simulink model "Channelizer"  (R2026a)
settings: Solver=VariableStepAuto  StopTime=1e-5
InitFcn:
  | init;
values from neighbouring files (symbols this model uses):
  ch0_en = 0    [channelizer_demo_init.m]    (also in init.m)
  ch0_qam = 0    [channelizer_demo_init.m]    (also in init.m)
  ch0_swp = 0    [channelizer_demo_init.m]    (also in init.m)
  ch10_en = 0    [channelizer_demo_init.m]    (also in init.m)
  ch10_qam = 0    [channelizer_demo_init.m]    (also in init.m)
  ch10_swp = 0    [channelizer_demo_init.m]    (also in init.m)
  ch11_en = 0    [channelizer_demo_init.m]    (also in init.m)
  ch11_qam = 0    [channelizer_demo_init.m]    (also in init.m)
  ch11_swp = 0    [channelizer_demo_init.m]    (also in init.m)
  ch12_en = 0    [channelizer_demo_init.m]    (also in init.m)
  ch12_qam = 0    [channelizer_demo_init.m]    (also in init.m)
  ch12_swp = 0    [channelizer_demo_init.m]    (also in init.m)
  ch13_en = 0    [channelizer_demo_init.m]    (also in init.m)
  ch13_qam = 0    [channelizer_demo_init.m]    (also in init.m)
  ch13_swp = 0    [channelizer_demo_init.m]    (also in init.m)
  ch14_en = 0    [channelizer_demo_init.m]    (also in init.m)
  ch14_qam = 0    [channelizer_demo_init.m]    (also in init.m)
  ch14_swp = 0    [channelizer_demo_init.m]    (also in init.m)
  ch15_en = 0    [channelizer_demo_init.m]    (also in init.m)
  ch15_qam = 0    [channelizer_demo_init.m]    (also in init.m)
  ch15_swp = 0    [channelizer_demo_init.m]    (also in init.m)
  ch1_en = 1    [channelizer_demo_init.m]    (also in init.m)
  ch1_qam = 0    [channelizer_demo_init.m]    (also in init.m)
  ch1_swp = 0    [channelizer_demo_init.m]    (also in init.m)
  ch2_en = 1    [channelizer_demo_init.m]    (also in init.m)
  ch2_qam = 0    [channelizer_demo_init.m]    (also in init.m)
  ch2_swp = 0    [channelizer_demo_init.m]    (also in init.m)
  ch3_en = 0    [channelizer_demo_init.m]    (also in init.m)
  ch3_qam = 0    [channelizer_demo_init.m]    (also in init.m)
  ch3_swp = 0    [channelizer_demo_init.m]    (also in init.m)
  ch4_en = 0    [channelizer_demo_init.m]    (also in init.m)
  ch4_qam = 0    [channelizer_demo_init.m]    (also in init.m)
  ch4_swp = 0    [channelizer_demo_init.m]    (also in init.m)
  ch5_en = 1    [channelizer_demo_init.m]    (also in init.m)
  ch5_qam = 1    [channelizer_demo_init.m]    (also in init.m)
  ch5_swp = 0    [channelizer_demo_init.m]    (also in init.m)
  ch6_en = 1    [channelizer_demo_init.m]    (also in init.m)
  ch6_qam = 1    [channelizer_demo_init.m]    (also in init.m)
  ch6_swp = 0    [channelizer_demo_init.m]    (also in init.m)
  ch7_en = 0    [channelizer_demo_init.m]    (also in init.m)
  ch7_qam = 0    [channelizer_demo_init.m]    (also in init.m)
  ch7_swp = 0    [channelizer_demo_init.m]    (also in init.m)
  ch8_en = 0    [channelizer_demo_init.m]    (also in init.m)
  ch8_qam = 0    [channelizer_demo_init.m]    (also in init.m)
  ch8_swp = 0    [channelizer_demo_init.m]    (also in init.m)
  ch9_en = 0    [channelizer_demo_init.m]    (also in init.m)
  ch9_qam = 0    [channelizer_demo_init.m]    (also in init.m)
  ch9_swp = 0    [channelizer_demo_init.m]    (also in init.m)
  ch_filt_coef = 28 * ch_filt_coef / sum(ch_filt_coef(:))    [init.m]
  N = 2*1024    (= 2048)    [hil.m]    (also in init.m = 256)
  nvar = 0.01    [init.m]
  randph = 2*pi*rand(16,1)    [init.m]
  spec1_ch = 1    [channelizer_demo_init.m]    (also in init.m)
  spec2_ch = 2    [channelizer_demo_init.m]    (also in init.m)
  spec3_ch = 5    [channelizer_demo_init.m]    (also in init.m)
  spec4_ch = 6    [channelizer_demo_init.m]    (also in init.m)
  swp_rate0 = 0    [channelizer_demo_init.m]    (also in init.m)
  swp_rate1 = 0    [channelizer_demo_init.m]    (also in init.m)
  swp_rate10 = 0    [channelizer_demo_init.m]    (also in init.m)
  swp_rate11 = 0    [channelizer_demo_init.m]    (also in init.m)
  swp_rate12 = 0    [channelizer_demo_init.m]    (also in init.m)
  swp_rate13 = 0    [channelizer_demo_init.m]    (also in init.m)
  swp_rate14 = 0    [channelizer_demo_init.m]    (also in init.m)
  swp_rate15 = 0    [channelizer_demo_init.m]    (also in init.m)
  swp_rate2 = 0    [channelizer_demo_init.m]    (also in init.m)
  swp_rate3 = 0    [channelizer_demo_init.m]    (also in init.m)
  swp_rate4 = 0    [channelizer_demo_init.m]    (also in init.m)
  swp_rate5 = 0    [channelizer_demo_init.m]    (also in init.m)
  swp_rate6 = 0    [channelizer_demo_init.m]    (also in init.m)
  swp_rate7 = 0    [channelizer_demo_init.m]    (also in init.m)
  swp_rate8 = 0    [channelizer_demo_init.m]    (also in init.m)
  swp_rate9 = 0    [channelizer_demo_init.m]    (also in init.m)
  Ts = 16*(7/4)/8.75e9    (= 3.2e-09)    [init.m]
undefined symbols (not defined in the file or in its folder): Asymmetric, jsin, S, vsva2197, xcvc1902
libraries: aieUtilities x20, aieBasic x7, hlsBasic x4, aieDSP x2, vmcUtilities x1
(part 2 of 3)

== system Channelizer/DUT/AIE_FilterBank_SSR ==
  In1 : Inport
  PLIO1 : aieBasic/PLIO  PlioWidth=64  PlioFreqSpec=on  PlioFreq=625  ColLocation=0  channel=0  blockJsonConstraints=[]  deprecateConstraints=0
  PLIO48 : aieBasic/PLIO  PlioWidth=64  PlioFreqSpec=on  PlioFreq=625  ColLocation=0  channel=0  blockJsonConstraints=[]  deprecateConstraints=0
  run_i1 : aieBasic/AIE Class Kernel  KernelAllAttrs=|  PortNames={'sig_i'; 'sig_o'}  PortSerializedTypes={'{Q2{P{Tinput_stream{1{t{Scint16}}}}}}'; '{Q2{P{Toutput_stream{1{t{Scint16}}}}}}'}  PortWindowSizes={0.000000000000000000e+00; 0.000000000000000000e+00}  PortWindowMargins={0.000000000000000000e+00; 0.000000000000000000e+00}  PortSynchronicities={'auto', 'auto'}  PortSignalSizes={0.000000000000000000e+00; 1.024000000000000000e+03}  ClassTemplateSpecKind=implicit  ClassTemplateParamNames={'pattern'; 'NSAMP'}  ClassTemplateParamKinds={'nontype'; 'nontype'}  ClassTemplateParamTypes={'unsigned int'; 'unsigned int'}  ClassTemplateParamValues={'0', '2048'}  ClassCtorParamNames={'taps0_i'; 'taps1_i'}  ClassCtorParamSerializedTypes={'{R{C{Bi16}64}}'; '{R{C{Bi16}64}}'}  ClassCtorParamValues={'[0;2;-4;6;-13;54;-178;1985;-20;88;-287;1822;-22;100;-326;1570;2042;6;-4;2;259;-80;23;-8;569;-166;49;-9;911;-248;74;-14;-19;93;-307;1256;-14;74;-248;911;-9;49;-166;569;-8;23;-80;259;1256;-307;93;-19;1570;-326;100;-22;1822;-287;88;-20;1985;-178;54;-13;-8;23;-80;259;0;2;-4;6;-13;54;-178;1985;-20;88;-287;1822;1985;-178;54;-13;2042;6;-4;2;259;-80;23;-8;569;-166;49;-9;-22;100;-326;1570;-19;93;-307;1256;-14;74;-248;911;-9;49;-166;569;911;-248;74;-14;1256;-307;93;-19;1570;-326;100;-22;1822;-287;88;-20;-9;49;-166;569;-8;23;-80;259;0;2;-4;6;-13;54;-178;1985;1822;-287;88;-20;1985;-178;54;-13;2042;6;-4;2;259;-80;23;-8;-20;88;-287;1822;-22;100;-326;1570;-19;93;-307;1256;-14;74;-248;911;569;-166;49;-9;911;-248;74;-14;1256;-307;93;-19;1570;-326;100;-22;-14;74;-248;911;-9;49;-166;569;-8;23;-80;259;0;2;-4;6;1570;-326;100;-22;1822;-287;88;-20;1985;-178;54;-13;2042;6;-4;2;-13;54;-178;1985;-20;88;-287;1822;-22;100;-326;1570;-19;93;-307;1256;259;-80;23;-8;569;-166;49;-9;911;-248;74;-14;1256;-307;93;-19;-19;93;-307;1256;-14;74;-248;911;-9;49;-166;569;-8;23;-80;259;1256;-307;93;-19;1570;-326;100;-22;1822;-287;88;-20;1985;-178;54;-13;0;2;-4;6;-13;54;-178;1985;-20;88;-287;1822;-22;100;-326;1570;2042;6;-4;2;259;-80;23;-8;569;-166;49;-9;911;-248;74;-14;-22;100;-326;1570;-19;93;-307;1256;-14;74;-248;911;-9;49;-166;569;911;-248;74;-14;1256;-307;93;-19;1570;-326;100;-22;1822;-287;88;-20;-8;23;-80;259;0;2;-4;6;-13;54;-178;1985;-20;88;-287;1822;1985;-178;54;-13;2042;6;-4;2;259;-80;23;-8;569;-166;49;-9;-20;88;-287;1822;-22;100;-326;1570;-19;93;-307;1256;-14;74;-248;911;569;-166;49;-9;911;-248;74;-14;1256;-307;93;-19;1570;-326;100;-22;-9;49;-166;569;-8;23;-80;259;0;2;-4;6;-13;54;-178;1985;1822;-287;88;-20;1985;-178;54;-13;2042;6;-4;2;259;-80;23;-8;-13;54;-178;1985;-20;88;-287;1822;-22;100;-326;1570;-19;93;-307;1256;259;-80;23;-8;569;-166;49;-9;911;-248;74;-14;1256;-307;93;-19;-14;74;-248;911;-9;49;-166;569;-8;23;-80;259;0;2;-4;6;1570;-326;100;-22;1822;-287;88;-20;1985;-178;54;-13;2042;6;-4;2]', '[6;12;-40;124;-6;28;-95;2027;-17;74;-241;1916;-22;97;-314;1706;2027;-95;28;-6;124;-40;12;6;408;-123;36;-8;737;-209;62;-12;-21;99;-322;1419;-17;85;-281;1085;-12;62;-209;737;-8;36;-123;408;1085;-281;85;-17;1419;-322;99;-21;1706;-314;97;-22;1916;-241;74;-17;-8;36;-123;408;6;12;-40;124;-6;28;-95;2027;-17;74;-241;1916;1916;-241;74;-17;2027;-95;28;-6;124;-40;12;6;408;-123;36;-8;-22;97;-314;1706;-21;99;-322;1419;-17;85;-281;1085;-12;62;-209;737;737;-209;62;-12;1085;-281;85;-17;1419;-322;99;-21;1706;-314;97;-22;-12;62;-209;737;-8;36;-123;408;6;12;-40;124;-6;28;-95;2027;1706;-314;97;-22;1916;-241;74;-17;2027;-95;28;-6;124;-40;12;6;-17;74;-241;1916;-22;97;-314;1706;-21;99;-322;1419;-17;85;-281;1085;408;-123;36;-8;737;-209;62;-12;1085;-281;85;-17;1419;-322;99;-21;-17;85;-281;1085;-12;62;-209;737;-8;36;-123;408;6;12;-40;124;1419;-322;99;-21;1706;-314;97;-22;1916;-241;74;-17;2027;-95;28;-6;-6;28;-95;2027;-17;74;-241;1916;-22;97;-314;1706;-21;99;-322;1419;124;-40;12;6;408;-123;36;-8;737;-209;62;-12;1085;-281;85;-17;-21;99;-322;1419;-17;85;-281;1085;-12;62;-209;737;-8;36;-123;408;1085;-281;85;-17;1419;-322;99;-21;1706;-314;97;-22;1916;-241;74;-17;6;12;-40;124;-6;28;-95;2027;-17;74;-241;1916;-22;97;-314;1706;2027;-95;28;-6;124;-40;12;6;408;-123;36;-8;737;-209;62;-12;-22;97;-314;1706;-21;99;-322;1419;-17;85;-281;1085;-12;62;-209;737;737;-209;62;-12;1085;-281;85;-17;1419;-322;99;-21;1706;-314;97;-22;-8;36;-123;408;6;12;-40;124;-6;28;-95;2027;-17;74;-241;1916;1916;-241;74;-17;2027;-95;28;-6;124;-40;12;6;408;-123;36;-8;-17;74;-241;1916;-22;97;-314;1706;-21;99;-322;1419;-17;85;-281;1085;408;-123;36;-8;737;-209;62;-12;1085;-281;85;-17;1419;-322;99;-21;-12;62;-209;737;-8;36;-123;408;6;12;-40;124;-6;28;-95;2027;1706;-314;97;-22;1916;-241;74;-17;2027;-95;28;-6;124;-40;12;6;-6;28;-95;2027;-17;74;-241;1916;-22;97;-314;1706;-21;99;-322;1419;124;-40;12;6;408;-123;36;-8;737;-209;62;-12;1085;-281;85;-17;-17;85;-281;1085;-12;62;-209;737;-8;36;-123;408;6;12;-40;124;1419;-322;99;-21;1706;-314;97;-22;1916;-241;74;-17;2027;-95;28;-6]'}  ClassIndex=1  ClassCtorIndex=1  ClassTabVisible=on  ClassTemplateParamsVisible=on  ClassCtorDeclVisible=on  ClassCtorParamsVisible=on  FunctionTabVisible=on  PreSSR=8  isImport=false  FunctionDecl=|  PortAttrs={ 'input', 'sig_i', 'input_stream_cint16 * restrict', '', '0', '', ''; 'output', 'sig_o', 'output_stream_cint16 * restrict', '', '', '', '4*N' }  PortAttrsEnables={'off', 'off', 'off', 'off', 'off', 'off', 'off';'off', 'off', 'off', 'off', 'off', 'off', 'on'}  SampleTime=-1  ClassDeclTypeOptions=C[1 1]@t74@template < unsigned int pattern, unsigned int NSAMP > class polyphase_fir;  ClassDecl=template < unsigned int pattern, unsigned int NSAMP > class polyphase_fir;  ClassTemplateParams={ 'pattern', 'unsigned int', '[0; 1; 2; 3; 4; 5; 6; 7]'; 'NSAMP', 'unsigned int', 'NSAMP' }  ClassTemplateParamsEnables={'off', 'off', 'on';'off', 'off', 'on'}  ClassCtorDeclTypeOptions=C[1 1]@t69@polyphase_fir(int16 ( & taps0_i ) [ 64 ], int16 ( & taps1_i ) [ 64 ])  ClassCtorDecl=polyphase_fir(int16 ( & taps0_i ) [ 64 ], int16 ( & taps1_i ) [ 64 ])  ClassCtorParams={ 'taps0_i', 'int16 ( &) [ 64 ]', '[tile0_tapsA; tile1_tapsA; tile2_tapsA; tile3_tapsA; tile4_tapsA; tile5_tapsA; tile6_tapsA; tile7_tapsA]'; 'taps1_i', 'int16 ( &) [ 64 ]', '[tile0_tapsB; tile1_tapsB; tile2_tapsB; tile3_tapsB; tile4_tapsB; tile5_tapsB; tile6_tapsB; tile7_tapsB]' }  KernelHeaderFile=aie/polyphase_fir.h  KernelClassName=polyphase_fir  KernelFunction=run_i  KernelSourceFile=aie/polyphase_fir.cpp  KernelSearchPaths={}  PreProcOptions={}  ssr=filterbank_ssr  blockJsonConstraints=[]
      KernelAllAttrs=|
      | s[12;12;9;9;19;14;21;23;21;23;24;21;15;17;12;24;26;26;26;27;28;9;21;23;23;23;24;25;14;19;19;29]@FunctionNameDeclFileNamePortNamesPortTypesPortSerializedTypesPortDirectionsPortWindowSizeEnablesPortWindowMarginEnablesPortBufferSizeEnablesPortBufferMarginEnablesPortSynchronicityEnablesPortSignalSizeEnablesPortBufferSizesPortBufferMarginsFunctionDeclFunctionTemplateSpecKindFunctionTemplateParamNamesFunctionTemplateParamKindsFunctionTemplateParamTypesFunctionTemplateParamValuesFunctionTemplateParamEnablesClassDeclClassTemplateSpecKindClassTemplateParamNamesClassTemplateParamKindsClassTemplateParamTypesClassTemplateParamValuesClassTemplateParamEnablesClassCtorDeclsClassCtorParamNamesClassCtorParamTypesClassCtorParamSerializedTypes[1 1]@C[32 1]@t5@run_it25@../../aie/polyphase_fir.hC[2 1]@t5@sig_it5@sig_oC[2 1]@t30@input_stream_cint16 * restrictt31@output_stream_cint16 * restrictC[2 1]@t37@{Q2{P{Tinput_stream{1{t{Scint16}}}}}}t38@{Q2{P{Toutput_stream{1{t{Scint16}}}}}}C[2 1]@t5@inputt6@outputC[2 1]@l0@l0@C[2 1]@l0@l0@C[2 1]@l0@l0@C[2 1]@l0@l0@C[2 1]@l0@l0@C[2 1]@l0@l1@C[2 1]@nnC[2 1]@nnt158@template < unsigned int pattern, unsigned int NSAMP > 
      | void polyphase_fir::
      | run_i(input_stream_cint16 * restrict sig_i, output_stream_cint16 * restrict sig_o)t4@nonee[0 1]@e[0 1]@e[0 1]@e[0 1]@e[0 1]@t74@template < unsigned int pattern, unsigned int NSAMP > class polyphase_fir;t8@implicitC[2 1]@t7@patternt5@NSAMPC[2 1]@t7@nontypet7@nontypeC[2 1]@t12@unsigned intt12@unsigned intC[2 1]@nnC[2 1]@l1@l1@C[1 1]@t69@polyphase_fir(int16 ( & taps0_i ) [ 64 ], int16 ( & taps1_i ) [ 64 ])C[1 1]@C[2 1]@t7@taps0_it7@taps1_iC[1 1]@C[2 1]@t17@int16 ( &) [ 64 ]t17@int16 ( &) [ 64 ]C[1 1]@C[2 1]@t14@{R{C{Bi16}64}}t14@{R{C{Bi16}64}}
      FunctionDecl=|
      | template < unsigned int pattern, unsigned int NSAMP > 
      | void polyphase_fir::
      | run_i(input_stream_cint16 * restrict sig_i, output_stream_cint16 * restrict sig_o)
  Out1 : Outport
  wires:
  run_i1/1 -> PLIO1/1
  PLIO1/1 -> Out1/1
  PLIO48/1 -> run_i1/1
  In1/1 -> PLIO48/1

== system Channelizer/Wideband_Signal/Random QAM ==
  Add : Sum
  Constant1 : Constant  SampleTime=-1
  Constant17 : Constant  SampleTime=-1
  Gain1 : Gain  Gain=2
  Gain7 : Gain  Gain=2
  Gain9 : Gain  Gain=1/sqrt(10)
  Product : Product
  Real-Imag to Complex : RealImagToComplex
  Round : Rounding  Operator=round
  Round1 : Rounding  Operator=round
  Selector : Selector  InputPortWidth=32*N  IndexOptions=Index vector (dialog)  Indices=1:2:32*N  OutputSizes=1
  Selector1 : Selector  InputPortWidth=32*N  IndexOptions=Index vector (dialog)  Indices=2:2:32*N  OutputSizes=1
  Subtract1 : Sum  Inputs=+-
  Uniform Random Number : UniformRandomNumber  Minimum=0  Seed=round(2^32*rand(32*N,1))  SampleTime=Ts*N  VectorParams1D=off
  Uniform Random Number2 : UniformRandomNumber  Minimum=0  Seed=round(2^32*rand(32*N,1))  SampleTime=Ts*N  VectorParams1D=off
  Out1 : Outport
  wires:
  Gain7/1 -> Add/1
  Constant17/1 -> Add/2
  Real-Imag to Complex/1 -> Out1/1
  Gain9/1 -> Selector1/1, Selector/1
  Selector/1 -> Real-Imag to Complex/1
  Selector1/1 -> Real-Imag to Complex/2
  Round/1 -> Gain7/1
  Uniform Random Number/1 -> Round/1
  Uniform Random Number2/1 -> Round1/1
  Constant1/1 -> Subtract1/2
  Gain1/1 -> Subtract1/1
  Round1/1 -> Gain1/1
  Product/1 -> Gain9/1
  Add/1 -> Product/1
  Subtract1/1 -> Product/2

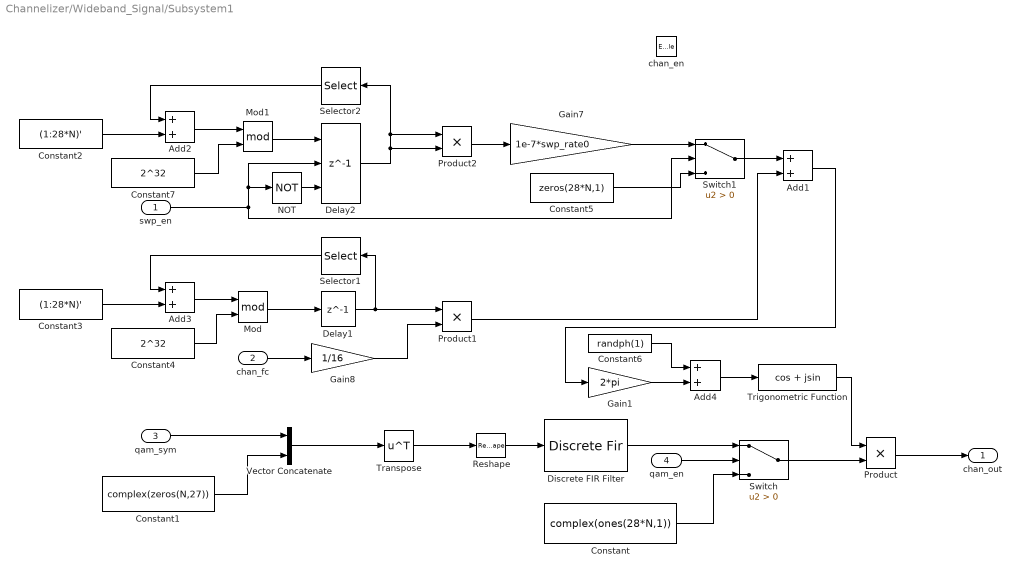
== system Channelizer/Wideband_Signal/Subsystem1 ==
  swp_en : Inport
  chan_fc : Inport  Port=2
  qam_sym : Inport  Port=3
  qam_en : Inport  Port=4
  chan_en : EnablePort
  Add{1..4} (4 alike) : Sum
  Constant : Constant  Value=complex(ones(28*N,1))  SampleTime=-1
  Constant1 : Constant  Value=complex(zeros(N,27))  VectorParams1D=off  SampleTime=-1
  Constant2 : Constant  Value=(1:28*N)'  SampleTime=-1
  Constant3 : Constant  Value=(1:28*N)'  SampleTime=-1
  Constant4 : Constant  Value=2^32  SampleTime=-1
  Constant5 : Constant  Value=zeros(28*N,1)  SampleTime=-1
  Constant6 : Constant  Value=randph(1)  SampleTime=-1
  Constant7 : Constant  Value=2^32  SampleTime=-1
  Delay1 : Delay  DelayLength=1  InitialCondition=(0:28*N-1)'
  Delay2 : Delay  DelayLength=1  InitialCondition=(1:28*N)'  ExternalReset=Falling  ShowEnablePort=on
      settings: InputPortMap=u0,e6,r5
  Discrete FIR Filter : DiscreteFir  Coefficients=ch_filt_coef  InputProcessing=Columns as channels (frame based)
  Gain1 : Gain  Gain=2*pi  OutDataTypeStr=double
  Gain7 : Gain  Gain=1e-7*swp_rate0  ParamDataTypeStr=double  OutDataTypeStr=double  SaturateOnIntegerOverflow=on
  Gain8 : Gain  Gain=1/16  OutDataTypeStr=double
  Mod : Math  Operator=mod
  Mod1 : Math  Operator=mod
  NOT : Logic  Operator=NOT  IconShape=distinctive  AllPortsSameDT=off  OutDataTypeStr=boolean
  Product : Product
  Product1 : Product
  Product2 : Product
  Reshape : Reshape
  Selector1 : Selector  InputPortWidth=28*N  IndexOptions=Index vector (dialog)  Indices=28*N  OutputSizes=1
  Selector2 : Selector  InputPortWidth=28*N  IndexOptions=Index vector (dialog)  Indices=28*N  OutputSizes=1
  Switch : Switch  Criteria=u2 > Threshold  SaturateOnIntegerOverflow=off  InputSameDT=off
  Switch1 : Switch  Criteria=u2 > Threshold  SaturateOnIntegerOverflow=off  InputSameDT=off
  Transpose : Math  Operator=transpose
  Trigonometric Function : Trigonometry  Operator=cos + jsin
  Vector Concatenate : Concatenate  Mode=Multidimensional array  ConcatenateDimension=2
  chan_out : Outport  OutputWhenDisabled=reset  InitialOutput=zeros(28*N,1)
  wires:
  Product/1 -> chan_out/1
  Switch/1 -> Product/2
  Discrete FIR Filter/1 -> Switch/1
  qam_en/1 -> Switch/2
  Constant/1 -> Switch/3
  Vector Concatenate/1 -> Transpose/1
  qam_sym/1 -> Vector Concatenate/1
  Constant1/1 -> Vector Concatenate/2
  Transpose/1 -> Reshape/1
  Reshape/1 -> Discrete FIR Filter/1
  Delay1/1 -> Product1/1, Selector1/1
  Selector1/1 -> Add3/1
  Constant3/1 -> Add3/2
  Mod/1 -> Delay1/1
  Add3/1 -> Mod/1
  Constant4/1 -> Mod/2
  Constant6/1 -> Add4/1
  Trigonometric Function/1 -> Product/1
  Add4/1 -> Trigonometric Function/1
  chan_fc/1 -> Gain8/1
  Gain8/1 -> Product1/2
  Gain1/1 -> Add4/2
  swp_en/1 -> NOT/1, Delay2/2, Switch1/2
  Constant5/1 -> Switch1/3
  Product2/1 -> Gain7/1
  Gain7/1 -> Switch1/1
  Switch1/1 -> Add1/1
  Product1/1 -> Add1/2
  Add1/1 -> Gain1/1
  Mod1/1 -> Delay2/1
  Constant2/1 -> Add2/2
  Selector2/1 -> Add2/1
  Delay2/1 -> Product2/1, Selector2/1, Product2/2
  Add2/1 -> Mod1/1
  Constant7/1 -> Mod1/2
  NOT/1 -> Delay2/3

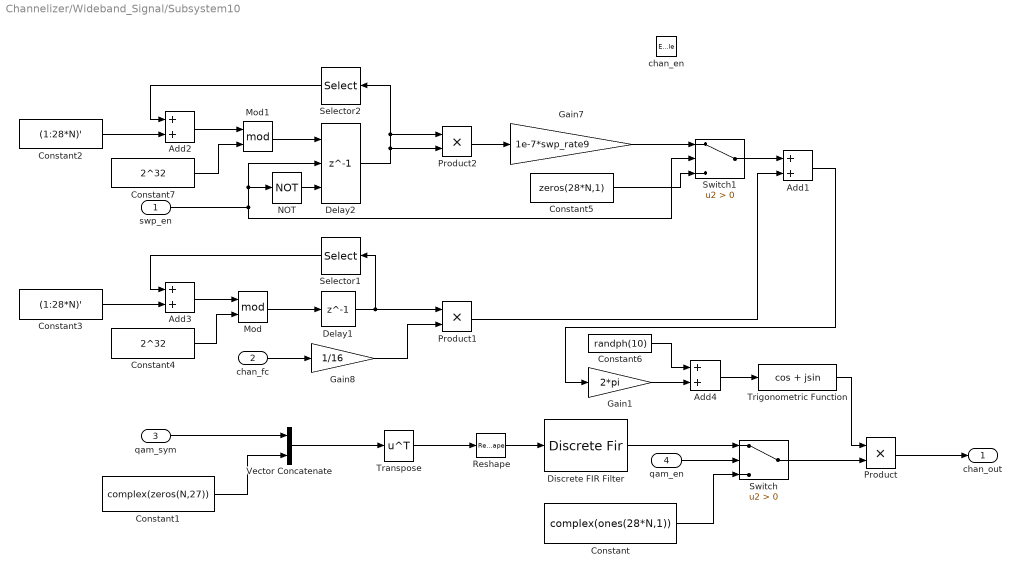
== system Channelizer/Wideband_Signal/Subsystem10 ==
  swp_en : Inport
  chan_fc : Inport  Port=2
  qam_sym : Inport  Port=3
  qam_en : Inport  Port=4
  chan_en : EnablePort
  Add{1..4} (4 alike) : Sum
  Constant : Constant  Value=complex(ones(28*N,1))  SampleTime=-1
  Constant1 : Constant  Value=complex(zeros(N,27))  VectorParams1D=off  SampleTime=-1
  Constant2 : Constant  Value=(1:28*N)'  SampleTime=-1
  Constant3 : Constant  Value=(1:28*N)'  SampleTime=-1
  Constant4 : Constant  Value=2^32  SampleTime=-1
  Constant5 : Constant  Value=zeros(28*N,1)  SampleTime=-1
  Constant6 : Constant  Value=randph(10)  SampleTime=-1
  Constant7 : Constant  Value=2^32  SampleTime=-1
  Delay1 : Delay  DelayLength=1  InitialCondition=(0:28*N-1)'
  Delay2 : Delay  DelayLength=1  InitialCondition=(1:28*N)'  ExternalReset=Falling  ShowEnablePort=on
      settings: InputPortMap=u0,e6,r5
  Discrete FIR Filter : DiscreteFir  Coefficients=ch_filt_coef  InputProcessing=Columns as channels (frame based)
  Gain1 : Gain  Gain=2*pi  OutDataTypeStr=double
  Gain7 : Gain  Gain=1e-7*swp_rate9  ParamDataTypeStr=double  OutDataTypeStr=double  SaturateOnIntegerOverflow=on
  Gain8 : Gain  Gain=1/16  OutDataTypeStr=double
  Mod : Math  Operator=mod
  Mod1 : Math  Operator=mod
  NOT : Logic  Operator=NOT  IconShape=distinctive  AllPortsSameDT=off  OutDataTypeStr=boolean
  Product : Product
  Product1 : Product
  Product2 : Product
  Reshape : Reshape
  Selector1 : Selector  InputPortWidth=28*N  IndexOptions=Index vector (dialog)  Indices=28*N  OutputSizes=1
  Selector2 : Selector  InputPortWidth=28*N  IndexOptions=Index vector (dialog)  Indices=28*N  OutputSizes=1
  Switch : Switch  Criteria=u2 > Threshold  SaturateOnIntegerOverflow=off  InputSameDT=off
  Switch1 : Switch  Criteria=u2 > Threshold  SaturateOnIntegerOverflow=off  InputSameDT=off
  Transpose : Math  Operator=transpose
  Trigonometric Function : Trigonometry  Operator=cos + jsin
  Vector Concatenate : Concatenate  Mode=Multidimensional array  ConcatenateDimension=2
  chan_out : Outport  OutputWhenDisabled=reset  InitialOutput=zeros(28*N,1)
  wires:
  Product/1 -> chan_out/1
  Switch/1 -> Product/2
  Discrete FIR Filter/1 -> Switch/1
  qam_en/1 -> Switch/2
  Constant/1 -> Switch/3
  Vector Concatenate/1 -> Transpose/1
  qam_sym/1 -> Vector Concatenate/1
  Constant1/1 -> Vector Concatenate/2
  Transpose/1 -> Reshape/1
  Reshape/1 -> Discrete FIR Filter/1
  Delay1/1 -> Product1/1, Selector1/1
  Selector1/1 -> Add3/1
  Constant3/1 -> Add3/2
  Mod/1 -> Delay1/1
  Add3/1 -> Mod/1
  Constant4/1 -> Mod/2
  Constant6/1 -> Add4/1
  Trigonometric Function/1 -> Product/1
  Add4/1 -> Trigonometric Function/1
  chan_fc/1 -> Gain8/1
  Gain8/1 -> Product1/2
  Gain1/1 -> Add4/2
  swp_en/1 -> NOT/1, Delay2/2, Switch1/2
  Constant5/1 -> Switch1/3
  Product2/1 -> Gain7/1
  Gain7/1 -> Switch1/1
  Switch1/1 -> Add1/1
  Product1/1 -> Add1/2
  Add1/1 -> Gain1/1
  Mod1/1 -> Delay2/1
  Constant2/1 -> Add2/2
  Selector2/1 -> Add2/1
  Delay2/1 -> Product2/1, Selector2/1, Product2/2
  Add2/1 -> Mod1/1
  Constant7/1 -> Mod1/2
  NOT/1 -> Delay2/3

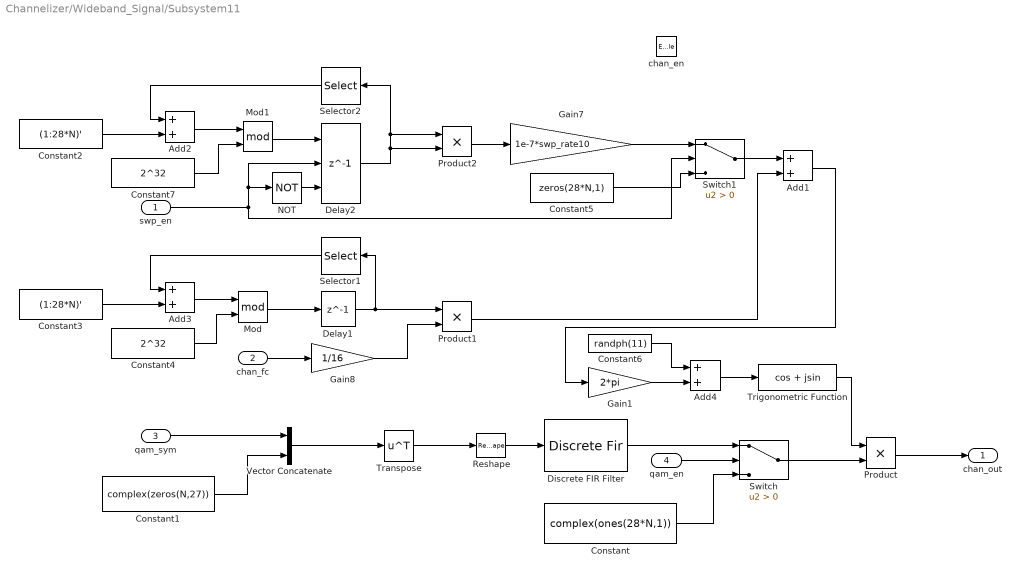
== system Channelizer/Wideband_Signal/Subsystem11 ==
  swp_en : Inport
  chan_fc : Inport  Port=2
  qam_sym : Inport  Port=3
  qam_en : Inport  Port=4
  chan_en : EnablePort
  Add{1..4} (4 alike) : Sum
  Constant : Constant  Value=complex(ones(28*N,1))  SampleTime=-1
  Constant1 : Constant  Value=complex(zeros(N,27))  VectorParams1D=off  SampleTime=-1
  Constant2 : Constant  Value=(1:28*N)'  SampleTime=-1
  Constant3 : Constant  Value=(1:28*N)'  SampleTime=-1
  Constant4 : Constant  Value=2^32  SampleTime=-1
  Constant5 : Constant  Value=zeros(28*N,1)  SampleTime=-1
  Constant6 : Constant  Value=randph(11)  SampleTime=-1
  Constant7 : Constant  Value=2^32  SampleTime=-1
  Delay1 : Delay  DelayLength=1  InitialCondition=(0:28*N-1)'
  Delay2 : Delay  DelayLength=1  InitialCondition=(1:28*N)'  ExternalReset=Falling  ShowEnablePort=on
      settings: InputPortMap=u0,e6,r5
  Discrete FIR Filter : DiscreteFir  Coefficients=ch_filt_coef  InputProcessing=Columns as channels (frame based)
  Gain1 : Gain  Gain=2*pi  OutDataTypeStr=double
  Gain7 : Gain  Gain=1e-7*swp_rate10  ParamDataTypeStr=double  OutDataTypeStr=double  SaturateOnIntegerOverflow=on
  Gain8 : Gain  Gain=1/16  OutDataTypeStr=double
  Mod : Math  Operator=mod
  Mod1 : Math  Operator=mod
  NOT : Logic  Operator=NOT  IconShape=distinctive  AllPortsSameDT=off  OutDataTypeStr=boolean
  Product : Product
  Product1 : Product
  Product2 : Product
  Reshape : Reshape
  Selector1 : Selector  InputPortWidth=28*N  IndexOptions=Index vector (dialog)  Indices=28*N  OutputSizes=1
  Selector2 : Selector  InputPortWidth=28*N  IndexOptions=Index vector (dialog)  Indices=28*N  OutputSizes=1
  Switch : Switch  Criteria=u2 > Threshold  SaturateOnIntegerOverflow=off  InputSameDT=off
  Switch1 : Switch  Criteria=u2 > Threshold  SaturateOnIntegerOverflow=off  InputSameDT=off
  Transpose : Math  Operator=transpose
  Trigonometric Function : Trigonometry  Operator=cos + jsin
  Vector Concatenate : Concatenate  Mode=Multidimensional array  ConcatenateDimension=2
  chan_out : Outport  OutputWhenDisabled=reset  InitialOutput=zeros(28*N,1)
  wires:
  Product/1 -> chan_out/1
  Switch/1 -> Product/2
  Discrete FIR Filter/1 -> Switch/1
  qam_en/1 -> Switch/2
  Constant/1 -> Switch/3
  Vector Concatenate/1 -> Transpose/1
  qam_sym/1 -> Vector Concatenate/1
  Constant1/1 -> Vector Concatenate/2
  Transpose/1 -> Reshape/1
  Reshape/1 -> Discrete FIR Filter/1
  Delay1/1 -> Product1/1, Selector1/1
  Selector1/1 -> Add3/1
  Constant3/1 -> Add3/2
  Mod/1 -> Delay1/1
  Add3/1 -> Mod/1
  Constant4/1 -> Mod/2
  Constant6/1 -> Add4/1
  Trigonometric Function/1 -> Product/1
  Add4/1 -> Trigonometric Function/1
  chan_fc/1 -> Gain8/1
  Gain8/1 -> Product1/2
  Gain1/1 -> Add4/2
  swp_en/1 -> NOT/1, Delay2/2, Switch1/2
  Constant5/1 -> Switch1/3
  Product2/1 -> Gain7/1
  Gain7/1 -> Switch1/1
  Switch1/1 -> Add1/1
  Product1/1 -> Add1/2
  Add1/1 -> Gain1/1
  Mod1/1 -> Delay2/1
  Constant2/1 -> Add2/2
  Selector2/1 -> Add2/1
  Delay2/1 -> Product2/1, Selector2/1, Product2/2
  Add2/1 -> Mod1/1
  Constant7/1 -> Mod1/2
  NOT/1 -> Delay2/3

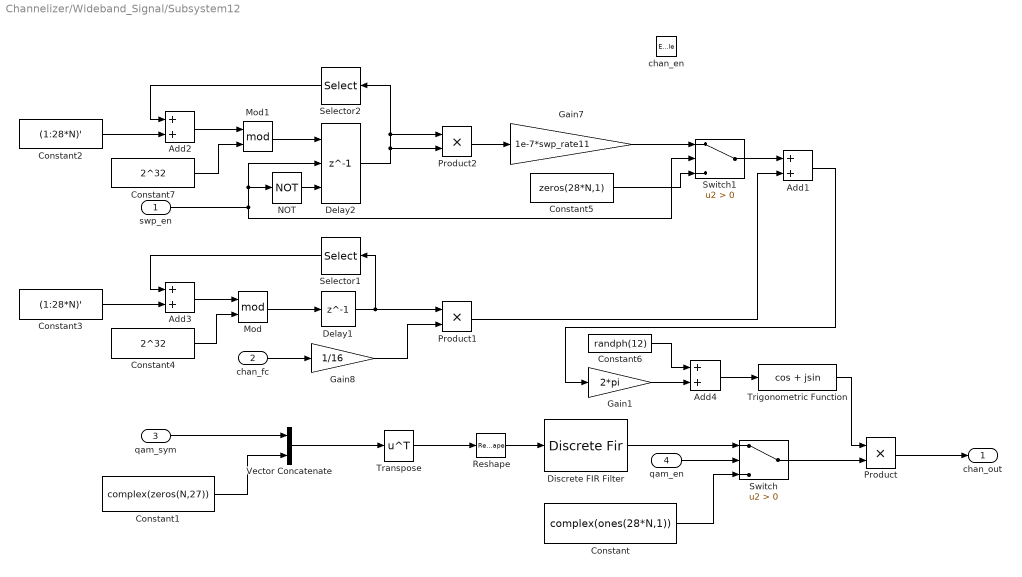
== system Channelizer/Wideband_Signal/Subsystem12 ==
  swp_en : Inport
  chan_fc : Inport  Port=2
  qam_sym : Inport  Port=3
  qam_en : Inport  Port=4
  chan_en : EnablePort
  Add{1..4} (4 alike) : Sum
  Constant : Constant  Value=complex(ones(28*N,1))  SampleTime=-1
  Constant1 : Constant  Value=complex(zeros(N,27))  VectorParams1D=off  SampleTime=-1
  Constant2 : Constant  Value=(1:28*N)'  SampleTime=-1
  Constant3 : Constant  Value=(1:28*N)'  SampleTime=-1
  Constant4 : Constant  Value=2^32  SampleTime=-1
  Constant5 : Constant  Value=zeros(28*N,1)  SampleTime=-1
  Constant6 : Constant  Value=randph(12)  SampleTime=-1
  Constant7 : Constant  Value=2^32  SampleTime=-1
  Delay1 : Delay  DelayLength=1  InitialCondition=(0:28*N-1)'
  Delay2 : Delay  DelayLength=1  InitialCondition=(1:28*N)'  ExternalReset=Falling  ShowEnablePort=on
      settings: InputPortMap=u0,e6,r5
  Discrete FIR Filter : DiscreteFir  Coefficients=ch_filt_coef  InputProcessing=Columns as channels (frame based)
  Gain1 : Gain  Gain=2*pi  OutDataTypeStr=double
  Gain7 : Gain  Gain=1e-7*swp_rate11  ParamDataTypeStr=double  OutDataTypeStr=double  SaturateOnIntegerOverflow=on
  Gain8 : Gain  Gain=1/16  OutDataTypeStr=double
  Mod : Math  Operator=mod
  Mod1 : Math  Operator=mod
  NOT : Logic  Operator=NOT  IconShape=distinctive  AllPortsSameDT=off  OutDataTypeStr=boolean
  Product : Product
  Product1 : Product
  Product2 : Product
  Reshape : Reshape
  Selector1 : Selector  InputPortWidth=28*N  IndexOptions=Index vector (dialog)  Indices=28*N  OutputSizes=1
  Selector2 : Selector  InputPortWidth=28*N  IndexOptions=Index vector (dialog)  Indices=28*N  OutputSizes=1
  Switch : Switch  Criteria=u2 > Threshold  SaturateOnIntegerOverflow=off  InputSameDT=off
  Switch1 : Switch  Criteria=u2 > Threshold  SaturateOnIntegerOverflow=off  InputSameDT=off
  Transpose : Math  Operator=transpose
  Trigonometric Function : Trigonometry  Operator=cos + jsin
  Vector Concatenate : Concatenate  Mode=Multidimensional array  ConcatenateDimension=2
  chan_out : Outport  OutputWhenDisabled=reset  InitialOutput=zeros(28*N,1)
  wires:
  Product/1 -> chan_out/1
  Switch/1 -> Product/2
  Discrete FIR Filter/1 -> Switch/1
  qam_en/1 -> Switch/2
  Constant/1 -> Switch/3
  Vector Concatenate/1 -> Transpose/1
  qam_sym/1 -> Vector Concatenate/1
  Constant1/1 -> Vector Concatenate/2
  Transpose/1 -> Reshape/1
  Reshape/1 -> Discrete FIR Filter/1
  Delay1/1 -> Product1/1, Selector1/1
  Selector1/1 -> Add3/1
  Constant3/1 -> Add3/2
  Mod/1 -> Delay1/1
  Add3/1 -> Mod/1
  Constant4/1 -> Mod/2
  Constant6/1 -> Add4/1
  Trigonometric Function/1 -> Product/1
  Add4/1 -> Trigonometric Function/1
  chan_fc/1 -> Gain8/1
  Gain8/1 -> Product1/2
  Gain1/1 -> Add4/2
  swp_en/1 -> NOT/1, Delay2/2, Switch1/2
  Constant5/1 -> Switch1/3
  Product2/1 -> Gain7/1
  Gain7/1 -> Switch1/1
  Switch1/1 -> Add1/1
  Product1/1 -> Add1/2
  Add1/1 -> Gain1/1
  Mod1/1 -> Delay2/1
  Constant2/1 -> Add2/2
  Selector2/1 -> Add2/1
  Delay2/1 -> Product2/1, Selector2/1, Product2/2
  Add2/1 -> Mod1/1
  Constant7/1 -> Mod1/2
  NOT/1 -> Delay2/3

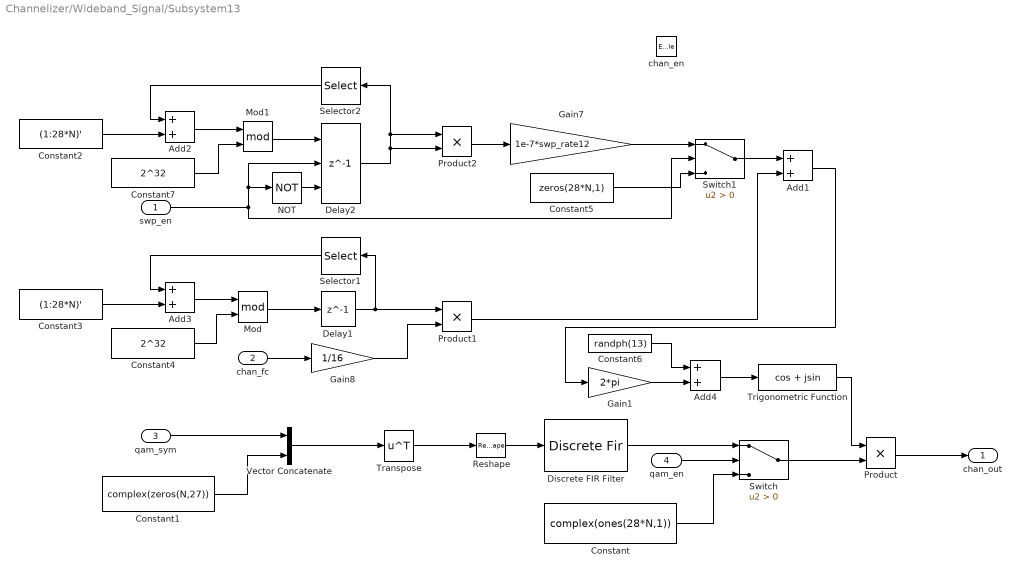
== system Channelizer/Wideband_Signal/Subsystem13 ==
  swp_en : Inport
  chan_fc : Inport  Port=2
  qam_sym : Inport  Port=3
  qam_en : Inport  Port=4
  chan_en : EnablePort
  Add{1..4} (4 alike) : Sum
  Constant : Constant  Value=complex(ones(28*N,1))  SampleTime=-1
  Constant1 : Constant  Value=complex(zeros(N,27))  VectorParams1D=off  SampleTime=-1
  Constant2 : Constant  Value=(1:28*N)'  SampleTime=-1
  Constant3 : Constant  Value=(1:28*N)'  SampleTime=-1
  Constant4 : Constant  Value=2^32  SampleTime=-1
  Constant5 : Constant  Value=zeros(28*N,1)  SampleTime=-1
  Constant6 : Constant  Value=randph(13)  SampleTime=-1
  Constant7 : Constant  Value=2^32  SampleTime=-1
  Delay1 : Delay  DelayLength=1  InitialCondition=(0:28*N-1)'
  Delay2 : Delay  DelayLength=1  InitialCondition=(1:28*N)'  ExternalReset=Falling  ShowEnablePort=on
      settings: InputPortMap=u0,e6,r5
  Discrete FIR Filter : DiscreteFir  Coefficients=ch_filt_coef  InputProcessing=Columns as channels (frame based)
  Gain1 : Gain  Gain=2*pi  OutDataTypeStr=double
  Gain7 : Gain  Gain=1e-7*swp_rate12  ParamDataTypeStr=double  OutDataTypeStr=double  SaturateOnIntegerOverflow=on
  Gain8 : Gain  Gain=1/16  OutDataTypeStr=double
  Mod : Math  Operator=mod
  Mod1 : Math  Operator=mod
  NOT : Logic  Operator=NOT  IconShape=distinctive  AllPortsSameDT=off  OutDataTypeStr=boolean
  Product : Product
  Product1 : Product
  Product2 : Product
  Reshape : Reshape
  Selector1 : Selector  InputPortWidth=28*N  IndexOptions=Index vector (dialog)  Indices=28*N  OutputSizes=1
  Selector2 : Selector  InputPortWidth=28*N  IndexOptions=Index vector (dialog)  Indices=28*N  OutputSizes=1
  Switch : Switch  Criteria=u2 > Threshold  SaturateOnIntegerOverflow=off  InputSameDT=off
  Switch1 : Switch  Criteria=u2 > Threshold  SaturateOnIntegerOverflow=off  InputSameDT=off
  Transpose : Math  Operator=transpose
  Trigonometric Function : Trigonometry  Operator=cos + jsin
  Vector Concatenate : Concatenate  Mode=Multidimensional array  ConcatenateDimension=2
  chan_out : Outport  OutputWhenDisabled=reset  InitialOutput=zeros(28*N,1)
  wires:
  Product/1 -> chan_out/1
  Switch/1 -> Product/2
  Discrete FIR Filter/1 -> Switch/1
  qam_en/1 -> Switch/2
  Constant/1 -> Switch/3
  Vector Concatenate/1 -> Transpose/1
  qam_sym/1 -> Vector Concatenate/1
  Constant1/1 -> Vector Concatenate/2
  Transpose/1 -> Reshape/1
  Reshape/1 -> Discrete FIR Filter/1
  Delay1/1 -> Product1/1, Selector1/1
  Selector1/1 -> Add3/1
  Constant3/1 -> Add3/2
  Mod/1 -> Delay1/1
  Add3/1 -> Mod/1
  Constant4/1 -> Mod/2
  Constant6/1 -> Add4/1
  Trigonometric Function/1 -> Product/1
  Add4/1 -> Trigonometric Function/1
  chan_fc/1 -> Gain8/1
  Gain8/1 -> Product1/2
  Gain1/1 -> Add4/2
  swp_en/1 -> NOT/1, Delay2/2, Switch1/2
  Constant5/1 -> Switch1/3
  Product2/1 -> Gain7/1
  Gain7/1 -> Switch1/1
  Switch1/1 -> Add1/1
  Product1/1 -> Add1/2
  Add1/1 -> Gain1/1
  Mod1/1 -> Delay2/1
  Constant2/1 -> Add2/2
  Selector2/1 -> Add2/1
  Delay2/1 -> Product2/1, Selector2/1, Product2/2
  Add2/1 -> Mod1/1
  Constant7/1 -> Mod1/2
  NOT/1 -> Delay2/3

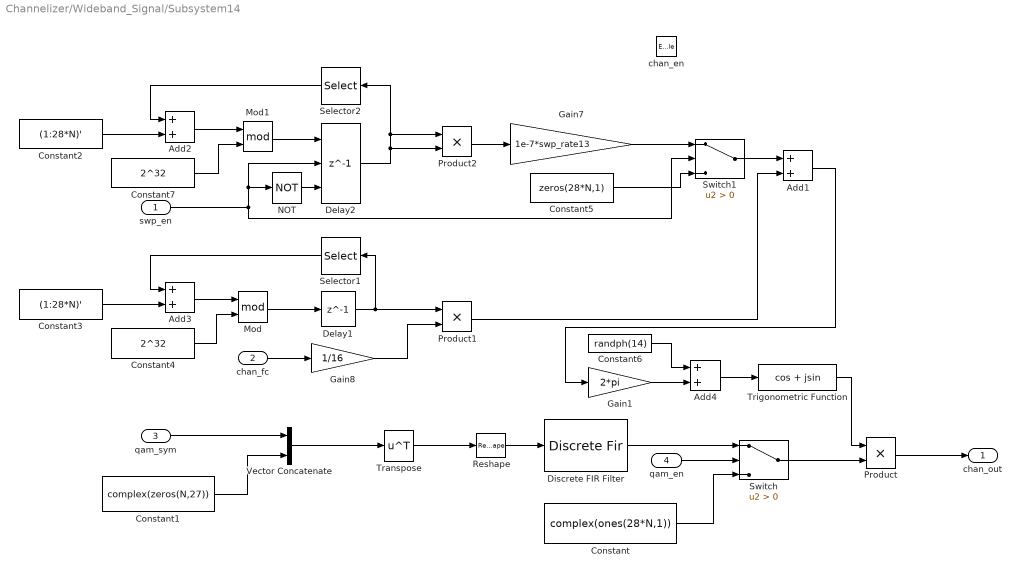
== system Channelizer/Wideband_Signal/Subsystem14 ==
  swp_en : Inport
  chan_fc : Inport  Port=2
  qam_sym : Inport  Port=3
  qam_en : Inport  Port=4
  chan_en : EnablePort
  Add{1..4} (4 alike) : Sum
  Constant : Constant  Value=complex(ones(28*N,1))  SampleTime=-1
  Constant1 : Constant  Value=complex(zeros(N,27))  VectorParams1D=off  SampleTime=-1
  Constant2 : Constant  Value=(1:28*N)'  SampleTime=-1
  Constant3 : Constant  Value=(1:28*N)'  SampleTime=-1
  Constant4 : Constant  Value=2^32  SampleTime=-1
  Constant5 : Constant  Value=zeros(28*N,1)  SampleTime=-1
  Constant6 : Constant  Value=randph(14)  SampleTime=-1
  Constant7 : Constant  Value=2^32  SampleTime=-1
  Delay1 : Delay  DelayLength=1  InitialCondition=(0:28*N-1)'
  Delay2 : Delay  DelayLength=1  InitialCondition=(1:28*N)'  ExternalReset=Falling  ShowEnablePort=on
      settings: InputPortMap=u0,e6,r5
  Discrete FIR Filter : DiscreteFir  Coefficients=ch_filt_coef  InputProcessing=Columns as channels (frame based)
  Gain1 : Gain  Gain=2*pi  OutDataTypeStr=double
  Gain7 : Gain  Gain=1e-7*swp_rate13  ParamDataTypeStr=double  OutDataTypeStr=double  SaturateOnIntegerOverflow=on
  Gain8 : Gain  Gain=1/16  OutDataTypeStr=double
  Mod : Math  Operator=mod
  Mod1 : Math  Operator=mod
  NOT : Logic  Operator=NOT  IconShape=distinctive  AllPortsSameDT=off  OutDataTypeStr=boolean
  Product : Product
  Product1 : Product
  Product2 : Product
  Reshape : Reshape
  Selector1 : Selector  InputPortWidth=28*N  IndexOptions=Index vector (dialog)  Indices=28*N  OutputSizes=1
  Selector2 : Selector  InputPortWidth=28*N  IndexOptions=Index vector (dialog)  Indices=28*N  OutputSizes=1
  Switch : Switch  Criteria=u2 > Threshold  SaturateOnIntegerOverflow=off  InputSameDT=off
  Switch1 : Switch  Criteria=u2 > Threshold  SaturateOnIntegerOverflow=off  InputSameDT=off
  Transpose : Math  Operator=transpose
  Trigonometric Function : Trigonometry  Operator=cos + jsin
  Vector Concatenate : Concatenate  Mode=Multidimensional array  ConcatenateDimension=2
  chan_out : Outport  OutputWhenDisabled=reset  InitialOutput=zeros(28*N,1)
  wires:
  Product/1 -> chan_out/1
  Switch/1 -> Product/2
  Discrete FIR Filter/1 -> Switch/1
  qam_en/1 -> Switch/2
  Constant/1 -> Switch/3
  Vector Concatenate/1 -> Transpose/1
  qam_sym/1 -> Vector Concatenate/1
  Constant1/1 -> Vector Concatenate/2
  Transpose/1 -> Reshape/1
  Reshape/1 -> Discrete FIR Filter/1
  Delay1/1 -> Product1/1, Selector1/1
  Selector1/1 -> Add3/1
  Constant3/1 -> Add3/2
  Mod/1 -> Delay1/1
  Add3/1 -> Mod/1
  Constant4/1 -> Mod/2
  Constant6/1 -> Add4/1
  Trigonometric Function/1 -> Product/1
  Add4/1 -> Trigonometric Function/1
  chan_fc/1 -> Gain8/1
  Gain8/1 -> Product1/2
  Gain1/1 -> Add4/2
  swp_en/1 -> NOT/1, Delay2/2, Switch1/2
  Constant5/1 -> Switch1/3
  Product2/1 -> Gain7/1
  Gain7/1 -> Switch1/1
  Switch1/1 -> Add1/1
  Product1/1 -> Add1/2
  Add1/1 -> Gain1/1
  Mod1/1 -> Delay2/1
  Constant2/1 -> Add2/2
  Selector2/1 -> Add2/1
  Delay2/1 -> Product2/1, Selector2/1, Product2/2
  Add2/1 -> Mod1/1
  Constant7/1 -> Mod1/2
  NOT/1 -> Delay2/3

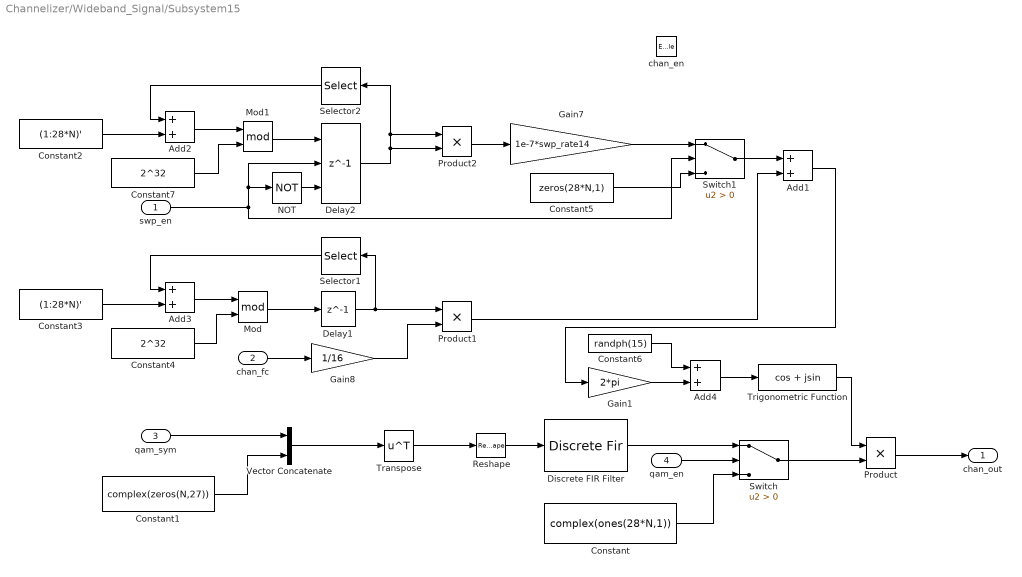
== system Channelizer/Wideband_Signal/Subsystem15 ==
  swp_en : Inport
  chan_fc : Inport  Port=2
  qam_sym : Inport  Port=3
  qam_en : Inport  Port=4
  chan_en : EnablePort
  Add{1..4} (4 alike) : Sum
  Constant : Constant  Value=complex(ones(28*N,1))  SampleTime=-1
  Constant1 : Constant  Value=complex(zeros(N,27))  VectorParams1D=off  SampleTime=-1
  Constant2 : Constant  Value=(1:28*N)'  SampleTime=-1
  Constant3 : Constant  Value=(1:28*N)'  SampleTime=-1
  Constant4 : Constant  Value=2^32  SampleTime=-1
  Constant5 : Constant  Value=zeros(28*N,1)  SampleTime=-1
  Constant6 : Constant  Value=randph(15)  SampleTime=-1
  Constant7 : Constant  Value=2^32  SampleTime=-1
  Delay1 : Delay  DelayLength=1  InitialCondition=(0:28*N-1)'
  Delay2 : Delay  DelayLength=1  InitialCondition=(1:28*N)'  ExternalReset=Falling  ShowEnablePort=on
      settings: InputPortMap=u0,e6,r5
  Discrete FIR Filter : DiscreteFir  Coefficients=ch_filt_coef  InputProcessing=Columns as channels (frame based)
  Gain1 : Gain  Gain=2*pi  OutDataTypeStr=double
  Gain7 : Gain  Gain=1e-7*swp_rate14  ParamDataTypeStr=double  OutDataTypeStr=double  SaturateOnIntegerOverflow=on
  Gain8 : Gain  Gain=1/16  OutDataTypeStr=double
  Mod : Math  Operator=mod
  Mod1 : Math  Operator=mod
  NOT : Logic  Operator=NOT  IconShape=distinctive  AllPortsSameDT=off  OutDataTypeStr=boolean
  Product : Product
  Product1 : Product
  Product2 : Product
  Reshape : Reshape
  Selector1 : Selector  InputPortWidth=28*N  IndexOptions=Index vector (dialog)  Indices=28*N  OutputSizes=1
  Selector2 : Selector  InputPortWidth=28*N  IndexOptions=Index vector (dialog)  Indices=28*N  OutputSizes=1
  Switch : Switch  Criteria=u2 > Threshold  SaturateOnIntegerOverflow=off  InputSameDT=off
  Switch1 : Switch  Criteria=u2 > Threshold  SaturateOnIntegerOverflow=off  InputSameDT=off
  Transpose : Math  Operator=transpose
  Trigonometric Function : Trigonometry  Operator=cos + jsin
  Vector Concatenate : Concatenate  Mode=Multidimensional array  ConcatenateDimension=2
  chan_out : Outport  OutputWhenDisabled=reset  InitialOutput=zeros(28*N,1)
  wires:
  Product/1 -> chan_out/1
  Switch/1 -> Product/2
  Discrete FIR Filter/1 -> Switch/1
  qam_en/1 -> Switch/2
  Constant/1 -> Switch/3
  Vector Concatenate/1 -> Transpose/1
  qam_sym/1 -> Vector Concatenate/1
  Constant1/1 -> Vector Concatenate/2
  Transpose/1 -> Reshape/1
  Reshape/1 -> Discrete FIR Filter/1
  Delay1/1 -> Product1/1, Selector1/1
  Selector1/1 -> Add3/1
  Constant3/1 -> Add3/2
  Mod/1 -> Delay1/1
  Add3/1 -> Mod/1
  Constant4/1 -> Mod/2
  Constant6/1 -> Add4/1
  Trigonometric Function/1 -> Product/1
  Add4/1 -> Trigonometric Function/1
  chan_fc/1 -> Gain8/1
  Gain8/1 -> Product1/2
  Gain1/1 -> Add4/2
  swp_en/1 -> NOT/1, Delay2/2, Switch1/2
  Constant5/1 -> Switch1/3
  Product2/1 -> Gain7/1
  Gain7/1 -> Switch1/1
  Switch1/1 -> Add1/1
  Product1/1 -> Add1/2
  Add1/1 -> Gain1/1
  Mod1/1 -> Delay2/1
  Constant2/1 -> Add2/2
  Selector2/1 -> Add2/1
  Delay2/1 -> Product2/1, Selector2/1, Product2/2
  Add2/1 -> Mod1/1
  Constant7/1 -> Mod1/2
  NOT/1 -> Delay2/3

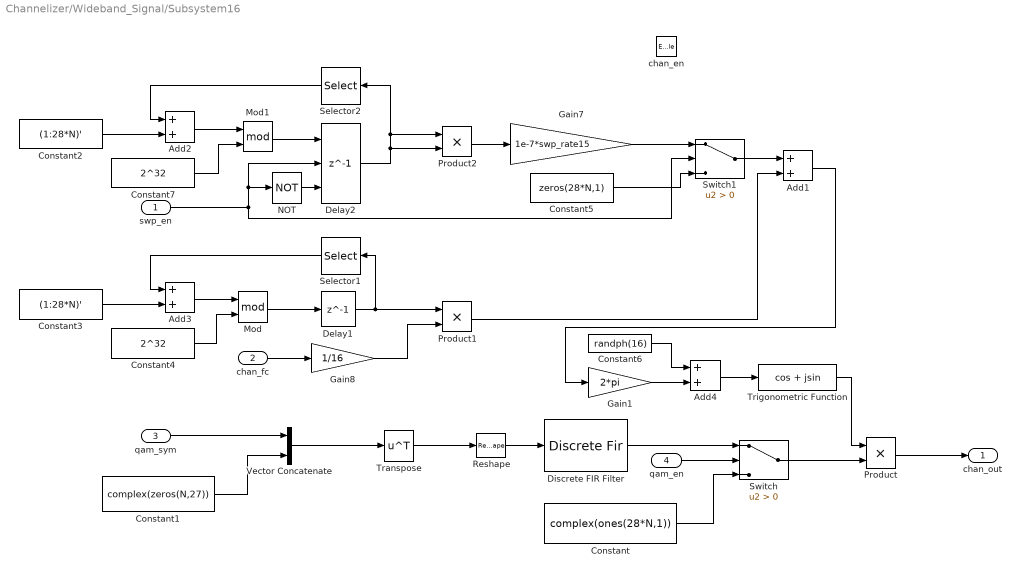
== system Channelizer/Wideband_Signal/Subsystem16 ==
  swp_en : Inport
  chan_fc : Inport  Port=2
  qam_sym : Inport  Port=3
  qam_en : Inport  Port=4
  chan_en : EnablePort
  Add{1..4} (4 alike) : Sum
  Constant : Constant  Value=complex(ones(28*N,1))  SampleTime=-1
  Constant1 : Constant  Value=complex(zeros(N,27))  VectorParams1D=off  SampleTime=-1
  Constant2 : Constant  Value=(1:28*N)'  SampleTime=-1
  Constant3 : Constant  Value=(1:28*N)'  SampleTime=-1
  Constant4 : Constant  Value=2^32  SampleTime=-1
  Constant5 : Constant  Value=zeros(28*N,1)  SampleTime=-1
  Constant6 : Constant  Value=randph(16)  SampleTime=-1
  Constant7 : Constant  Value=2^32  SampleTime=-1
  Delay1 : Delay  DelayLength=1  InitialCondition=(0:28*N-1)'
  Delay2 : Delay  DelayLength=1  InitialCondition=(1:28*N)'  ExternalReset=Falling  ShowEnablePort=on
      settings: InputPortMap=u0,e6,r5
  Discrete FIR Filter : DiscreteFir  Coefficients=ch_filt_coef  InputProcessing=Columns as channels (frame based)
  Gain1 : Gain  Gain=2*pi  OutDataTypeStr=double
  Gain7 : Gain  Gain=1e-7*swp_rate15  ParamDataTypeStr=double  OutDataTypeStr=double  SaturateOnIntegerOverflow=on
  Gain8 : Gain  Gain=1/16  OutDataTypeStr=double
  Mod : Math  Operator=mod
  Mod1 : Math  Operator=mod
  NOT : Logic  Operator=NOT  IconShape=distinctive  AllPortsSameDT=off  OutDataTypeStr=boolean
  Product : Product
  Product1 : Product
  Product2 : Product
  Reshape : Reshape
  Selector1 : Selector  InputPortWidth=28*N  IndexOptions=Index vector (dialog)  Indices=28*N  OutputSizes=1
  Selector2 : Selector  InputPortWidth=28*N  IndexOptions=Index vector (dialog)  Indices=28*N  OutputSizes=1
  Switch : Switch  Criteria=u2 > Threshold  SaturateOnIntegerOverflow=off  InputSameDT=off
  Switch1 : Switch  Criteria=u2 > Threshold  SaturateOnIntegerOverflow=off  InputSameDT=off
  Transpose : Math  Operator=transpose
  Trigonometric Function : Trigonometry  Operator=cos + jsin
  Vector Concatenate : Concatenate  Mode=Multidimensional array  ConcatenateDimension=2
  chan_out : Outport  OutputWhenDisabled=reset  InitialOutput=zeros(28*N,1)
  wires:
  Product/1 -> chan_out/1
  Switch/1 -> Product/2
  Discrete FIR Filter/1 -> Switch/1
  qam_en/1 -> Switch/2
  Constant/1 -> Switch/3
  Vector Concatenate/1 -> Transpose/1
  qam_sym/1 -> Vector Concatenate/1
  Constant1/1 -> Vector Concatenate/2
  Transpose/1 -> Reshape/1
  Reshape/1 -> Discrete FIR Filter/1
  Delay1/1 -> Product1/1, Selector1/1
  Selector1/1 -> Add3/1
  Constant3/1 -> Add3/2
  Mod/1 -> Delay1/1
  Add3/1 -> Mod/1
  Constant4/1 -> Mod/2
  Constant6/1 -> Add4/1
  Trigonometric Function/1 -> Product/1
  Add4/1 -> Trigonometric Function/1
  chan_fc/1 -> Gain8/1
  Gain8/1 -> Product1/2
  Gain1/1 -> Add4/2
  swp_en/1 -> NOT/1, Delay2/2, Switch1/2
  Constant5/1 -> Switch1/3
  Product2/1 -> Gain7/1
  Gain7/1 -> Switch1/1
  Switch1/1 -> Add1/1
  Product1/1 -> Add1/2
  Add1/1 -> Gain1/1
  Mod1/1 -> Delay2/1
  Constant2/1 -> Add2/2
  Selector2/1 -> Add2/1
  Delay2/1 -> Product2/1, Selector2/1, Product2/2
  Add2/1 -> Mod1/1
  Constant7/1 -> Mod1/2
  NOT/1 -> Delay2/3

== system Channelizer/Wideband_Signal/Subsystem2 ==
  swp_en : Inport
  chan_fc : Inport  Port=2
  qam_sym : Inport  Port=3
  qam_en : Inport  Port=4
  chan_en : EnablePort
  Add{1..4} (4 alike) : Sum
  Constant : Constant  Value=complex(ones(28*N,1))  SampleTime=-1
  Constant1 : Constant  Value=complex(zeros(N,27))  VectorParams1D=off  SampleTime=-1
  Constant2 : Constant  Value=(1:28*N)'  SampleTime=-1
  Constant3 : Constant  Value=(1:28*N)'  SampleTime=-1
  Constant4 : Constant  Value=2^32  SampleTime=-1
  Constant5 : Constant  Value=zeros(28*N,1)  SampleTime=-1
  Constant6 : Constant  Value=randph(2)  SampleTime=-1
  Constant7 : Constant  Value=2^32  SampleTime=-1
  Delay1 : Delay  DelayLength=1  InitialCondition=(0:28*N-1)'
  Delay2 : Delay  DelayLength=1  InitialCondition=(1:28*N)'  ExternalReset=Falling  ShowEnablePort=on
      settings: InputPortMap=u0,e6,r5
  Discrete FIR Filter : DiscreteFir  Coefficients=ch_filt_coef  InputProcessing=Columns as channels (frame based)
  Gain1 : Gain  Gain=2*pi  OutDataTypeStr=double
  Gain7 : Gain  Gain=1e-7*swp_rate1  ParamDataTypeStr=double  OutDataTypeStr=double  SaturateOnIntegerOverflow=on
  Gain8 : Gain  Gain=1/16  OutDataTypeStr=double
  Mod : Math  Operator=mod
  Mod1 : Math  Operator=mod
  NOT : Logic  Operator=NOT  IconShape=distinctive  AllPortsSameDT=off  OutDataTypeStr=boolean
  Product : Product
  Product1 : Product
  Product2 : Product
  Reshape : Reshape
  Selector1 : Selector  InputPortWidth=28*N  IndexOptions=Index vector (dialog)  Indices=28*N  OutputSizes=1
  Selector2 : Selector  InputPortWidth=28*N  IndexOptions=Index vector (dialog)  Indices=28*N  OutputSizes=1
  Switch : Switch  Criteria=u2 > Threshold  SaturateOnIntegerOverflow=off  InputSameDT=off
  Switch1 : Switch  Criteria=u2 > Threshold  SaturateOnIntegerOverflow=off  InputSameDT=off
  Transpose : Math  Operator=transpose
  Trigonometric Function : Trigonometry  Operator=cos + jsin
  Vector Concatenate : Concatenate  Mode=Multidimensional array  ConcatenateDimension=2
  chan_out : Outport  OutputWhenDisabled=reset  InitialOutput=zeros(28*N,1)
  wires:
  Product/1 -> chan_out/1
  Switch/1 -> Product/2
  Discrete FIR Filter/1 -> Switch/1
  qam_en/1 -> Switch/2
  Constant/1 -> Switch/3
  Vector Concatenate/1 -> Transpose/1
  qam_sym/1 -> Vector Concatenate/1
  Constant1/1 -> Vector Concatenate/2
  Transpose/1 -> Reshape/1
  Reshape/1 -> Discrete FIR Filter/1
  Delay1/1 -> Product1/1, Selector1/1
  Selector1/1 -> Add3/1
  Constant3/1 -> Add3/2
  Mod/1 -> Delay1/1
  Add3/1 -> Mod/1
  Constant4/1 -> Mod/2
  Constant6/1 -> Add4/1
  Trigonometric Function/1 -> Product/1
  Add4/1 -> Trigonometric Function/1
  chan_fc/1 -> Gain8/1
  Gain8/1 -> Product1/2
  Gain1/1 -> Add4/2
  swp_en/1 -> NOT/1, Delay2/2, Switch1/2
  Constant5/1 -> Switch1/3
  Product2/1 -> Gain7/1
  Gain7/1 -> Switch1/1
  Switch1/1 -> Add1/1
  Product1/1 -> Add1/2
  Add1/1 -> Gain1/1
  Mod1/1 -> Delay2/1
  Constant2/1 -> Add2/2
  Selector2/1 -> Add2/1
  Delay2/1 -> Product2/1, Selector2/1, Product2/2
  Add2/1 -> Mod1/1
  Constant7/1 -> Mod1/2
  NOT/1 -> Delay2/3

== system Channelizer/Wideband_Signal/Subsystem3 ==
  swp_en : Inport
  chan_fc : Inport  Port=2
  qam_sym : Inport  Port=3
  qam_en : Inport  Port=4
  chan_en : EnablePort
  Add{1..4} (4 alike) : Sum
  Constant : Constant  Value=complex(ones(28*N,1))  SampleTime=-1
  Constant1 : Constant  Value=complex(zeros(N,27))  VectorParams1D=off  SampleTime=-1
  Constant2 : Constant  Value=(1:28*N)'  SampleTime=-1
  Constant3 : Constant  Value=(1:28*N)'  SampleTime=-1
  Constant4 : Constant  Value=2^32  SampleTime=-1
  Constant5 : Constant  Value=zeros(28*N,1)  SampleTime=-1
  Constant6 : Constant  Value=randph(3)  SampleTime=-1
  Constant7 : Constant  Value=2^32  SampleTime=-1
  Delay1 : Delay  DelayLength=1  InitialCondition=(0:28*N-1)'
  Delay2 : Delay  DelayLength=1  InitialCondition=(1:28*N)'  ExternalReset=Falling  ShowEnablePort=on
      settings: InputPortMap=u0,e6,r5
  Discrete FIR Filter : DiscreteFir  Coefficients=ch_filt_coef  InputProcessing=Columns as channels (frame based)
  Gain1 : Gain  Gain=2*pi  OutDataTypeStr=double
  Gain7 : Gain  Gain=1e-7*swp_rate2  ParamDataTypeStr=double  OutDataTypeStr=double  SaturateOnIntegerOverflow=on
  Gain8 : Gain  Gain=1/16  OutDataTypeStr=double
  Mod : Math  Operator=mod
  Mod1 : Math  Operator=mod
  NOT : Logic  Operator=NOT  IconShape=distinctive  AllPortsSameDT=off  OutDataTypeStr=boolean
  Product : Product
  Product1 : Product
  Product2 : Product
  Reshape : Reshape
  Selector1 : Selector  InputPortWidth=28*N  IndexOptions=Index vector (dialog)  Indices=28*N  OutputSizes=1
  Selector2 : Selector  InputPortWidth=28*N  IndexOptions=Index vector (dialog)  Indices=28*N  OutputSizes=1
  Switch : Switch  Criteria=u2 > Threshold  SaturateOnIntegerOverflow=off  InputSameDT=off
  Switch1 : Switch  Criteria=u2 > Threshold  SaturateOnIntegerOverflow=off  InputSameDT=off
  Transpose : Math  Operator=transpose
  Trigonometric Function : Trigonometry  Operator=cos + jsin
  Vector Concatenate : Concatenate  Mode=Multidimensional array  ConcatenateDimension=2
  chan_out : Outport  OutputWhenDisabled=reset  InitialOutput=zeros(28*N,1)
  wires:
  Product/1 -> chan_out/1
  Switch/1 -> Product/2
  Discrete FIR Filter/1 -> Switch/1
  qam_en/1 -> Switch/2
  Constant/1 -> Switch/3
  Vector Concatenate/1 -> Transpose/1
  qam_sym/1 -> Vector Concatenate/1
  Constant1/1 -> Vector Concatenate/2
  Transpose/1 -> Reshape/1
  Reshape/1 -> Discrete FIR Filter/1
  Delay1/1 -> Product1/1, Selector1/1
  Selector1/1 -> Add3/1
  Constant3/1 -> Add3/2
  Mod/1 -> Delay1/1
  Add3/1 -> Mod/1
  Constant4/1 -> Mod/2
  Constant6/1 -> Add4/1
  Trigonometric Function/1 -> Product/1
  Add4/1 -> Trigonometric Function/1
  chan_fc/1 -> Gain8/1
  Gain8/1 -> Product1/2
  Gain1/1 -> Add4/2
  swp_en/1 -> NOT/1, Delay2/2, Switch1/2
  Constant5/1 -> Switch1/3
  Product2/1 -> Gain7/1
  Gain7/1 -> Switch1/1
  Switch1/1 -> Add1/1
  Product1/1 -> Add1/2
  Add1/1 -> Gain1/1
  Mod1/1 -> Delay2/1
  Constant2/1 -> Add2/2
  Selector2/1 -> Add2/1
  Delay2/1 -> Product2/1, Selector2/1, Product2/2
  Add2/1 -> Mod1/1
  Constant7/1 -> Mod1/2
  NOT/1 -> Delay2/3

== system Channelizer/Wideband_Signal/Subsystem4 ==
  swp_en : Inport
  chan_fc : Inport  Port=2
  qam_sym : Inport  Port=3
  qam_en : Inport  Port=4
  chan_en : EnablePort
  Add{1..4} (4 alike) : Sum
  Constant : Constant  Value=complex(ones(28*N,1))  SampleTime=-1
  Constant1 : Constant  Value=complex(zeros(N,27))  VectorParams1D=off  SampleTime=-1
  Constant2 : Constant  Value=(1:28*N)'  SampleTime=-1
  Constant3 : Constant  Value=(1:28*N)'  SampleTime=-1
  Constant4 : Constant  Value=2^32  SampleTime=-1
  Constant5 : Constant  Value=zeros(28*N,1)  SampleTime=-1
  Constant6 : Constant  Value=randph(4)  SampleTime=-1
  Constant7 : Constant  Value=2^32  SampleTime=-1
  Delay1 : Delay  DelayLength=1  InitialCondition=(0:28*N-1)'
  Delay2 : Delay  DelayLength=1  InitialCondition=(1:28*N)'  ExternalReset=Falling  ShowEnablePort=on
      settings: InputPortMap=u0,e6,r5
  Discrete FIR Filter : DiscreteFir  Coefficients=ch_filt_coef  InputProcessing=Columns as channels (frame based)
  Gain1 : Gain  Gain=2*pi  OutDataTypeStr=double
  Gain7 : Gain  Gain=1e-7*swp_rate3  ParamDataTypeStr=double  OutDataTypeStr=double  SaturateOnIntegerOverflow=on
  Gain8 : Gain  Gain=1/16  OutDataTypeStr=double
  Mod : Math  Operator=mod
  Mod1 : Math  Operator=mod
  NOT : Logic  Operator=NOT  IconShape=distinctive  AllPortsSameDT=off  OutDataTypeStr=boolean
  Product : Product
  Product1 : Product
  Product2 : Product
  Reshape : Reshape
  Selector1 : Selector  InputPortWidth=28*N  IndexOptions=Index vector (dialog)  Indices=28*N  OutputSizes=1
  Selector2 : Selector  InputPortWidth=28*N  IndexOptions=Index vector (dialog)  Indices=28*N  OutputSizes=1
  Switch : Switch  Criteria=u2 > Threshold  SaturateOnIntegerOverflow=off  InputSameDT=off
  Switch1 : Switch  Criteria=u2 > Threshold  SaturateOnIntegerOverflow=off  InputSameDT=off
  Transpose : Math  Operator=transpose
  Trigonometric Function : Trigonometry  Operator=cos + jsin
  Vector Concatenate : Concatenate  Mode=Multidimensional array  ConcatenateDimension=2
  chan_out : Outport  OutputWhenDisabled=reset  InitialOutput=zeros(28*N,1)
  wires:
  Product/1 -> chan_out/1
  Switch/1 -> Product/2
  Discrete FIR Filter/1 -> Switch/1
  qam_en/1 -> Switch/2
  Constant/1 -> Switch/3
  Vector Concatenate/1 -> Transpose/1
  qam_sym/1 -> Vector Concatenate/1
  Constant1/1 -> Vector Concatenate/2
  Transpose/1 -> Reshape/1
  Reshape/1 -> Discrete FIR Filter/1
  Delay1/1 -> Product1/1, Selector1/1
  Selector1/1 -> Add3/1
  Constant3/1 -> Add3/2
  Mod/1 -> Delay1/1
  Add3/1 -> Mod/1
  Constant4/1 -> Mod/2
  Constant6/1 -> Add4/1
  Trigonometric Function/1 -> Product/1
  Add4/1 -> Trigonometric Function/1
  chan_fc/1 -> Gain8/1
  Gain8/1 -> Product1/2
  Gain1/1 -> Add4/2
  swp_en/1 -> NOT/1, Delay2/2, Switch1/2
  Constant5/1 -> Switch1/3
  Product2/1 -> Gain7/1
  Gain7/1 -> Switch1/1
  Switch1/1 -> Add1/1
  Product1/1 -> Add1/2
  Add1/1 -> Gain1/1
  Mod1/1 -> Delay2/1
  Constant2/1 -> Add2/2
  Selector2/1 -> Add2/1
  Delay2/1 -> Product2/1, Selector2/1, Product2/2
  Add2/1 -> Mod1/1
  Constant7/1 -> Mod1/2
  NOT/1 -> Delay2/3
